simulink model "zad1"  (R2020b)
settings: Solver=FixedStepDiscrete  StartTime=0.0  StopTime=0.0  RelTol=1e-3
libraries: CPOiS_SourcesSinks x6, CPOiS_LinearTransforms x2, CPOiS_HistogramOperations x2, CPOiS_DataManipulation_DataTypeConversion x2, CPOiS_General x1
settings Model: Creator=jrybarz  LastModifiedBy=jrybarz

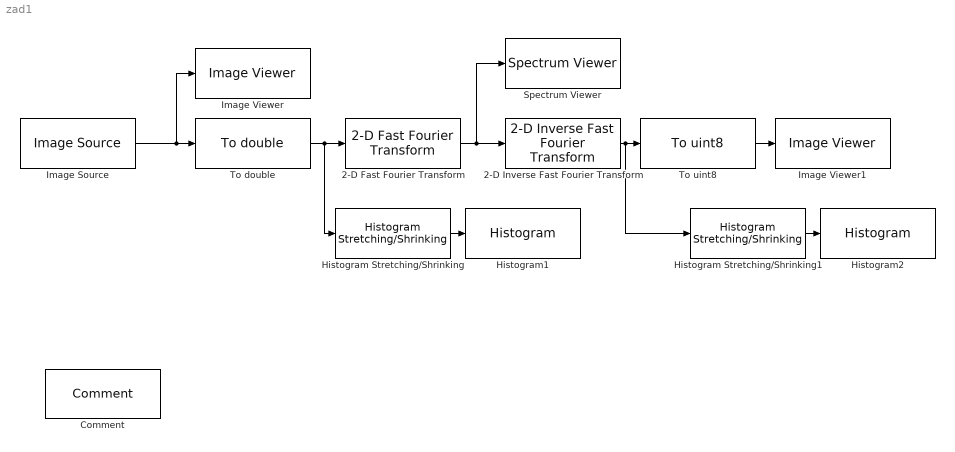
== system zad1 ==
  2-D Fast Fourier Transform : CPOiS_LinearTransforms/2-D Fast Fourier Transform
      settings: SourceProductName=CPOiS - Digital image and signal processing
  2-D Inverse Fast Fourier Transform : CPOiS_LinearTransforms/2-D Inverse Fast  Fourier Transform
      settings: SourceProductName=CPOiS - Digital image and signal processing
  Comment : CPOiS_General/Comment
      settings: SourceProductName=CPOiS - Digital image and signal processing
  Histogram Stretching/Shrinking : CPOiS_HistogramOperations/Histogram Stretching//Shrinking  minimum=0  maximum=255
      settings: SourceProductName=CPOiS - Digital image and signal processing
  Histogram Stretching/Shrinking1 : CPOiS_HistogramOperations/Histogram Stretching//Shrinking  minimum=0  maximum=255
      settings: SourceProductName=CPOiS - Digital image and signal processing
  Histogram1 : CPOiS_SourcesSinks/Histogram
      settings: SourceProductName=CPOiS - Digital image and signal processing
  Histogram2 : CPOiS_SourcesSinks/Histogram
      settings: SourceProductName=CPOiS - Digital image and signal processing
  Image Source : CPOiS_SourcesSinks/Image Source  FileSelection=marine.png
      settings: SourceProductName=CPOiS - Digital image and signal processing
  Image Viewer : CPOiS_SourcesSinks/Image Viewer
      settings: SourceProductName=CPOiS - Digital image and signal processing
  Image Viewer1 : CPOiS_SourcesSinks/Image Viewer
      settings: SourceProductName=CPOiS - Digital image and signal processing
  Spectrum Viewer : CPOiS_SourcesSinks/Spectrum Viewer
      settings: SourceProductName=CPOiS - Digital image and signal processing
  To double : CPOiS_DataManipulation_DataTypeConversion/To double
      settings: SourceProductName=CPOiS - Digital image and signal processing
  To uint8 : CPOiS_DataManipulation_DataTypeConversion/To uint8
      settings: SourceProductName=CPOiS - Digital image and signal processing
  wires:
  Image Source/1 -> Image Viewer/1, To double/1
  To double/1 -> Histogram Stretching/Shrinking/1, 2-D Fast Fourier Transform/1
  2-D Fast Fourier Transform/1 -> Spectrum Viewer/1, 2-D Inverse Fast Fourier Transform/1
  2-D Inverse Fast Fourier Transform/1 -> Histogram Stretching/Shrinking1/1, To uint8/1
  To uint8/1 -> Image Viewer1/1
  Histogram Stretching/Shrinking/1 -> Histogram1/1
  Histogram Stretching/Shrinking1/1 -> Histogram2/1
